simulink library "libTFActuatorCalc"  (R2020b)
settings: Solver=VariableStepAuto  StartTime=0.0  StopTime=10.0  RelTol=1e-3
settings Model: Creator=caatay  LastModifiedBy=caatay

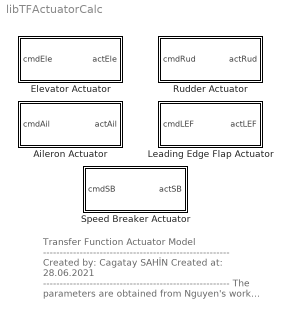
== system libTFActuatorCalc ==
  note: Transfer Function Actuator Model
      | --------------------------------------------------------
      | Created by: Cagatay SAHİN
      | Created at: 28.06.2021
      | --------------------------------------------------------
      | The parameters are obtained from Nguyen's
      | work and time constant parameters are
      | obtained from Steven's work
      | The references can be found in "references
      | folder".
      | --------------------------------------------------------
      | for question:
      | cagataysahin44@gmail.com
  Aileron Actuator : Subsystem  mask(Flight Control System Model - Actuator Model - Transfer Function Aileron Actuator Model Library){ail=outputs.trim.controls.aileron, cmd_ail_upper_limit=21.5, cmd_ail_lower_limit=-21.5, rate_ail_upper_limit=80, rate_ail_lower_limit=-80, ail_timeCons=20.2}
      mask prompts: ail "Trimmed Aileron Command"; cmd_ail_upper_limit "Upper Aileron Command Limit"; cmd_ail_lower_limit "Lower Aileron Command Limit"; rate_ail_upper_limit "Upper Aileron Rate Limit"; rate_ail_lower_limit "Lower Aileron Rate Limit"; ail_timeCons "Time Constant"
      mask help: Actuator Model with using basic transfer function and feedback methodology.
      mask Help:
      | This block calculates actuated aileron signal with using transfer function (feedback) methodology. Constants are obtained from Nguyen's paper and Steven's textbook.
      | -------------------------------------------------------------------------------------------------------------------------------------------------
      | Inputs of this block set are;
      | 	commanded_aileron = Commanded aileron deflection value that comes flight control system. [deg]
      | Output of this block set is;
      | 	actuated_aileron = Actuated aileron deflection value that comes actuator system. [deg]
      | -------------------------------------------------------------------------------------------------------------------------------------------------
      | Constants and some parameters are obtained from Nguyen's and Steven's work. Reference can be found in "literature" subfolder.
      | For question: "cagataysahin44@gmail.com"
      mask Display:
      | port_label('input',1,'\delta_{ail_{cmd}}','texmode','on');
      | 
      | port_label('output',1,'\delta_{ail_{act}}','texmode','on')
  Elevator Actuator : Subsystem  mask(Flight Control System Model - Actuator Model - Transfer Function Elevator Actuator Model Library){ele=outputs.trim.controls.elevator, cmd_ele_upper_limit=25, cmd_ele_lower_limit=-25, rate_ele_upper_limit=60, rate_ele_lower_limit=-60, ele_timeCons=20.2}
      mask prompts: ele "Trimmed Elevator Command"; cmd_ele_upper_limit "Upper Elevator Command Limit"; cmd_ele_lower_limit "Lower Elevator Command Limit"; rate_ele_upper_limit "Upper Elevator Rate Limit"; rate_ele_lower_limit "Lower Elevator Rate Limit"; ele_timeCons "Time Constant"
      mask help: Actuator Model with using basic transfer function and feedback methodology.
      mask Help:
      | This block calculates actuated elevator signal with using transfer function (feedback) methodology. Constants are obtained from Nguyen's paper and Steven's textbook.
      | -------------------------------------------------------------------------------------------------------------------------------------------------
      | Inputs of this block set are;
      | 	commanded_elevator = Commanded elevator deflection value that comes flight control system. [deg]
      | Output of this block set is;
      | 	actuated_elevator = Actuated elevator deflection value that comes actuator system. [deg]
      | -------------------------------------------------------------------------------------------------------------------------------------------------
      | Constants and some parameters are obtained from Nguyen's and Steven's work. Reference can be found in "literature" subfolder.
      | For question: "cagataysahin44@gmail.com"
      mask Display:
      | port_label('input',1,'\delta_{ele_{cmd}}','texmode','on');
      | 
      | port_label('output',1,'\delta_{ele_{act}}','texmode','on')
  Leading Edge Flap Actuator : Subsystem  mask(Flight Control System Model - Actuator Model - Transfer Function Leading Edge Flap Actuator Model Library){lef=outputs.trim.controls.lef, cmd_lef_upper_limit=25, cmd_lef_lower_limit=0, rate_lef_upper_limit=25, rate_lef_lower_limit=-25, lef_timeCons=1/0.136}
      mask prompts: lef "Trimmed LEF Command"; cmd_lef_upper_limit "Upper LEF Command Limit"; cmd_lef_lower_limit "Lower LEF Command Limit"; rate_lef_upper_limit "Upper LEF Rate Limit"; rate_lef_lower_limit "Lower LEF Rate Limit"; lef_timeCons "Time Constant"
      mask help: Actuator Model with using basic transfer function and feedback methodology.
      mask Help:
      | This block calculates actuated lef signal with using transfer function (feedback) methodology. Constants are obtained from Nguyen's paper and Steven's textbook.
      | -------------------------------------------------------------------------------------------------------------------------------------------------
      | Inputs of this block set are;
      | 	commanded_lef = Commanded lef deflection value that comes flight control system. [deg]
      | Output of this block set is;
      | 	actuated_lef= Actuated lef deflection value that comes actuator system. [deg]
      | -------------------------------------------------------------------------------------------------------------------------------------------------
      | Constants and some parameters are obtained from Nguyen's and Steven's work. Reference can be found in "literature" subfolder.
      | For question: "cagataysahin44@gmail.com"
      mask Display:
      | port_label('input',1,'\delta_{lef_{cmd}}','texmode','on');
      | 
      | port_label('output',1,'\delta_{lef_{act}}','texmode','on')
  Rudder Actuator : Subsystem  mask(Flight Control System Model - Actuator Model - Transfer Function Rudder Actuator Model Library){rud=outputs.trim.controls.rudder, cmd_rud_upper_limit=30, cmd_rud_lower_limit=-30, rate_rud_upper_limit=120, rate_rud_lower_limit=-120, rud_timeCons=20.2}
      mask prompts: rud "Trimmed Rudder Command"; cmd_rud_upper_limit "Upper Rodder Command Limit"; cmd_rud_lower_limit "Lower Rodder Command Limit"; rate_rud_upper_limit "Upper Rodder Rate Limit"; rate_rud_lower_limit "Lower Rodder Rate Limit"; rud_timeCons "Time Constant"
      mask help: Actuator Model with using basic transfer function and feedback methodology.
      mask Help:
      | This block calculates actuated rudder signal with using transfer function (feedback) methodology. Constants are obtained from Nguyen's paper and Steven's textbook.
      | -------------------------------------------------------------------------------------------------------------------------------------------------
      | Inputs of this block set are;
      | 	commanded_erudder = Commanded rudder deflection value that comes flight control system. [deg]
      | Output of this block set is;
      | 	actuated_rudder= Actuated rudder deflection value that comes actuator system. [deg]
      | -------------------------------------------------------------------------------------------------------------------------------------------------
      | Constants and some parameters are obtained from Nguyen's and Steven's work. Reference can be found in "literature" subfolder.
      | For question: "cagataysahin44@gmail.com"
      mask Display:
      | port_label('input',1,'\delta_{rud_{cmd}}','texmode','on');
      | 
      | port_label('output',1,'\delta_{rud_{act}}','texmode','on')
  Speed Breaker Actuator : Subsystem  mask(Flight Control System Model - Actuator Model - Transfer Function Speed Breaker Actuator Model Library){sb=outputs.trim.controls.sb, cmd_sb_upper_limit=60, cmd_sb_lower_limit=0, rate_sb_upper_limit=60, rate_sb_lower_limit=-60, sb_timeCons=20.2}
      mask prompts: sb "Trimmed LEF Command"; cmd_sb_upper_limit "Upper SB Command Limit"; cmd_sb_lower_limit "Lower SB Command Limit"; rate_sb_upper_limit "Upper SB Rate Limit"; rate_sb_lower_limit "Lower SB Rate Limit"; sb_timeCons "Time Constant"
      mask help: Actuator Model with using basic transfer function and feedback methodology.
      mask Help:
      | This block calculates actuated speed breaker signal with using transfer function (feedback) methodology. Constants are obtained from Nguyen's paper and Steven's textbook.
      | -------------------------------------------------------------------------------------------------------------------------------------------------
      | Inputs of this block set are;
      | 	commanded_sb = Commanded sb deflection value that comes flight control system. [deg]
      | Output of this block set is;
      | 	actuated_sb = Actuated sb deflection value that comes actuator system. [deg]
      | -------------------------------------------------------------------------------------------------------------------------------------------------
      | Constants and some parameters are obtained from Nguyen's and Steven's work. Reference can be found in "literature" subfolder.
      | For question: "cagataysahin44@gmail.com"
      mask Display:
      | port_label('input',1,'\delta_{sb_{cmd}}','texmode','on');
      | 
      | port_label('output',1,'\delta_{sb_{act}}','texmode','on')

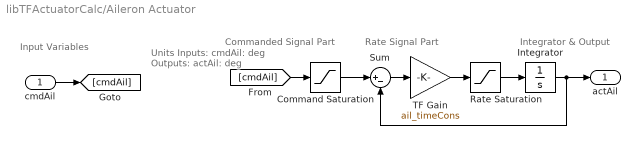
== system libTFActuatorCalc/Aileron Actuator ==
  note: Rate Signal Part
  note: Integrator & Output
  note: Input Variables
  note: Commanded Signal Part
  note: Units
      | Inputs:
      | cmdAil: deg
      | Outputs:
      | actAil: deg
  cmdAil : Inport
  Command Saturation : Saturate  UpperLimit=cmd_ail_upper_limit  LowerLimit=cmd_ail_lower_limit
  Integrator : Integrator  InitialCondition=ail
  Rate Saturation : Saturate  UpperLimit=rate_ail_upper_limit  LowerLimit=rate_ail_lower_limit
  Sum : Sum  Inputs=|+-
  TF Gain : Gain  Gain=ail_timeCons
  actAil : Outport  VectorParamsAs1DForOutWhenUnconnected=off
  wires:
  Sum/1 -> TF Gain/1
  TF Gain/1 -> Rate Saturation/1
  Command Saturation/1 -> Sum/1
  [cmdAil] -> Command Saturation/1
  cmdAil/1 -> [cmdAil]
  Integrator/1 -> Sum/2, actAil/1
  Rate Saturation/1 -> Integrator/1

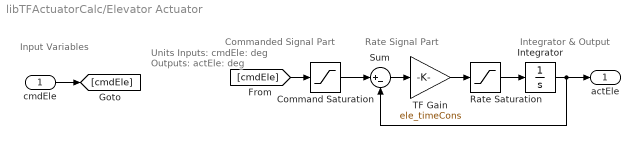
== system libTFActuatorCalc/Elevator Actuator ==
  note: Integrator & Output
  note: Rate Signal Part
  note: Commanded Signal Part
  note: Units
      | Inputs:
      | cmdEle: deg
      | Outputs:
      | actEle: deg
  note: Input Variables
  cmdEle : Inport
  Command Saturation : Saturate  UpperLimit=cmd_ele_upper_limit  LowerLimit=cmd_ele_lower_limit
  Integrator : Integrator  InitialCondition=ele
  Rate Saturation : Saturate  UpperLimit=rate_ele_upper_limit  LowerLimit=rate_ele_lower_limit
  Sum : Sum  Inputs=|+-
  TF Gain : Gain  Gain=ele_timeCons
  actEle : Outport  VectorParamsAs1DForOutWhenUnconnected=off
  wires:
  cmdEle/1 -> [cmdEle]
  Command Saturation/1 -> Sum/1
  [cmdEle] -> Command Saturation/1
  Sum/1 -> TF Gain/1
  Rate Saturation/1 -> Integrator/1
  Integrator/1 -> Sum/2, actEle/1
  TF Gain/1 -> Rate Saturation/1

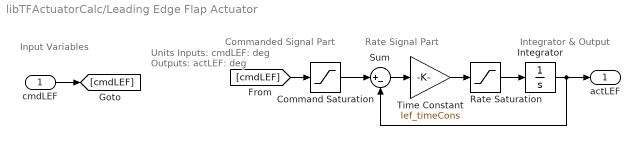
== system libTFActuatorCalc/Leading Edge Flap Actuator ==
  note: Commanded Signal Part
  note: Input Variables
  note: Units
      | Inputs:
      | cmdLEF: deg
      | Outputs:
      | actLEF: deg
  note: Integrator & Output
  note: Rate Signal Part
  cmdLEF : Inport
  Command Saturation : Saturate  UpperLimit=cmd_lef_upper_limit  LowerLimit=cmd_lef_lower_limit
  Integrator : Integrator  InitialCondition=lef
  Rate Saturation : Saturate  UpperLimit=rate_lef_upper_limit  LowerLimit=rate_lef_lower_limit
  Sum : Sum  Inputs=|+-
  Time Constant : Gain  Gain=lef_timeCons
  actLEF : Outport  VectorParamsAs1DForOutWhenUnconnected=off
  wires:
  Integrator/1 -> Sum/2, actLEF/1
  [cmdLEF] -> Command Saturation/1
  Rate Saturation/1 -> Integrator/1
  Command Saturation/1 -> Sum/1
  Sum/1 -> Time Constant/1
  cmdLEF/1 -> [cmdLEF]
  Time Constant/1 -> Rate Saturation/1

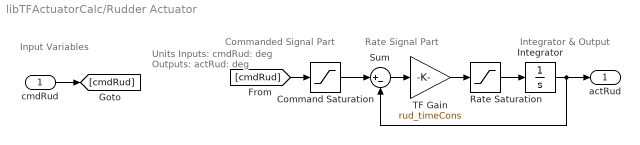
== system libTFActuatorCalc/Rudder Actuator ==
  note: Rate Signal Part
  note: Integrator & Output
  note: Input Variables
  note: Commanded Signal Part
  note: Units
      | Inputs:
      | cmdRud: deg
      | Outputs:
      | actRud: deg
  cmdRud : Inport
  Command Saturation : Saturate  UpperLimit=cmd_rud_upper_limit  LowerLimit=cmd_rud_lower_limit
  Integrator : Integrator  InitialCondition=rud
  Rate Saturation : Saturate  UpperLimit=rate_rud_upper_limit  LowerLimit=rate_rud_lower_limit
  Sum : Sum  Inputs=|+-
  TF Gain : Gain  Gain=rud_timeCons
  actRud : Outport  VectorParamsAs1DForOutWhenUnconnected=off
  wires:
  Sum/1 -> TF Gain/1
  TF Gain/1 -> Rate Saturation/1
  Command Saturation/1 -> Sum/1
  [cmdRud] -> Command Saturation/1
  cmdRud/1 -> [cmdRud]
  Integrator/1 -> Sum/2, actRud/1
  Rate Saturation/1 -> Integrator/1

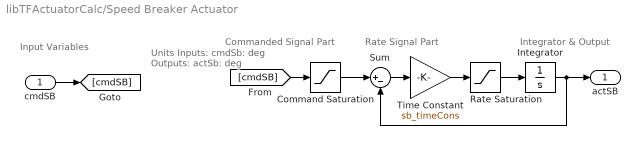
== system libTFActuatorCalc/Speed Breaker Actuator ==
  note: Rate Signal Part
  note: Commanded Signal Part
  note: Input Variables
  note: Units
      | Inputs:
      | cmdSb: deg
      | Outputs:
      | actSb: deg
  note: Integrator & Output
  cmdSB : Inport
  Command Saturation : Saturate  UpperLimit=cmd_sb_upper_limit  LowerLimit=cmd_sb_lower_limit
  Integrator : Integrator  InitialCondition=sb
  Rate Saturation : Saturate  UpperLimit=rate_sb_upper_limit  LowerLimit=rate_sb_lower_limit
  Sum : Sum  Inputs=|+-
  Time Constant : Gain  Gain=sb_timeCons
  actSB : Outport  VectorParamsAs1DForOutWhenUnconnected=off
  wires:
  cmdSB/1 -> [cmdSB]
  Rate Saturation/1 -> Integrator/1
  [cmdSB] -> Command Saturation/1
  Command Saturation/1 -> Sum/1
  Sum/1 -> Time Constant/1
  Integrator/1 -> Sum/2, actSB/1
  Time Constant/1 -> Rate Saturation/1
